simulink model "qpsk"  (R2015a)
settings: Solver=ode4  SolverMode=SingleTasking  StartTime=0.0  StopTime=Inf  RelTol=1e-3
libraries: dspsrcs4 x4, simulink x3, commrandsrc2 x1, commutil2 x1
settings Model: Creator=Artyom  LastModifiedBy=Artyom
settings OptimizationCC: BlockReduction=off  BooleanDataType=off
settings DebuggingCC: SaveWithParameterizedLinksMsg=none  UnderspecifiedInitializationDetection=Classic  MergeDetectMultiDrivingBlocksExec=none  SignalResolutionControl=TryResolveAllWithWarning
settings HardwareCC: TargetLongLongMode=on  TargetIntDivRoundTo=Zero  TargetEndianess=LittleEndian  TargetHWDeviceType=MATLAB Host  ProdEqTarget=off

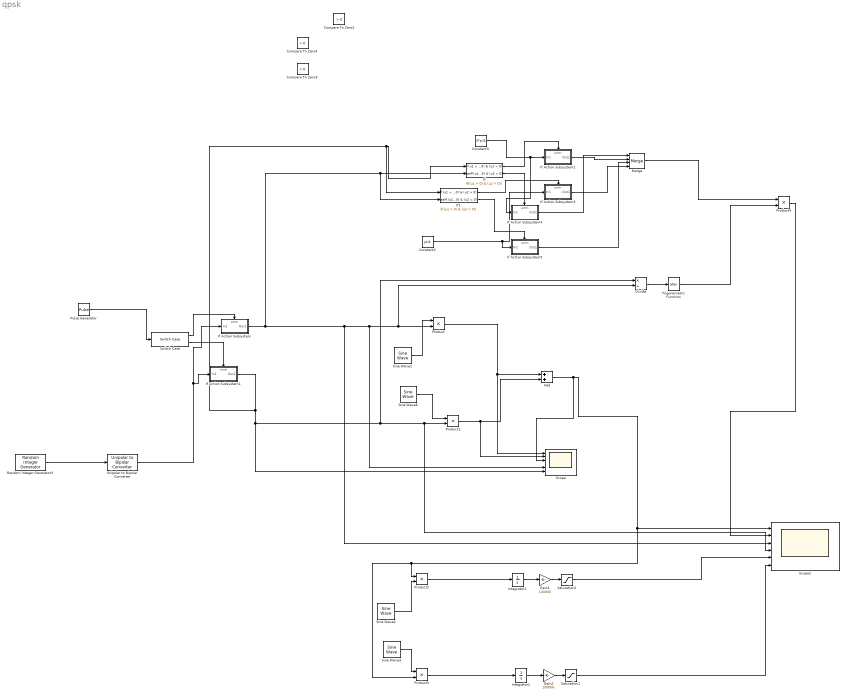
== system qpsk ==
  Add : Sum
  Compare To Zero2 : simulink/Logic and Bit Operations/Compare To Zero  relop=>  OutDataTypeStr=boolean
  Compare To Zero3 : simulink/Logic and Bit Operations/Compare To Zero  relop=<  OutDataTypeStr=boolean
  Compare To Zero4 : simulink/Logic and Bit Operations/Compare To Zero  relop=>  OutDataTypeStr=boolean
  Constant2 : Constant  Value=pi/4
  Constant3 : Constant  Value=3*pi/4
  Divide : Product  Inputs=*/
  Gain1 : Gain  Gain=100000
  Gain2 : Gain  Gain=100000
  If : If  NumInputs=2  IfExpression=(u1 < 0) & (u2 < 0)  ElseIfExpressions=(u1 < 0) & (u2 > 0)  ShowElse=off
  If Action Subsystem : Subsystem  TreatAsAtomicUnit=on
  If Action Subsystem1 : Subsystem  TreatAsAtomicUnit=on
  If Action Subsystem2 : Subsystem  TreatAsAtomicUnit=on
  If Action Subsystem3 : Subsystem  TreatAsAtomicUnit=on
  If Action Subsystem4 : Subsystem  TreatAsAtomicUnit=on
  If Action Subsystem5 : Subsystem  TreatAsAtomicUnit=on
  If1 : If  NumInputs=2  IfExpression=(u1 > 0) & (u2 > 0)  ElseIfExpressions=(u1 > 0) & (u2 < 0)  ShowElse=off
  Integrator1 : Integrator  LimitOutput=on  UpperSaturationLimit=0.00001  LowerSaturationLimit=-0.00001  ShowStatePort=on
  Integrator2 : Integrator  LimitOutput=on  UpperSaturationLimit=0.00001  LowerSaturationLimit=-0.00001  ShowStatePort=on
  Merge : Merge  Inputs=4
  Product : Product  OutDataTypeStr=Inherit: Same as first input
  Product{1..4} (4 alike) : Product
  Pulse Generator : DiscretePulseGenerator  PulseType=Time based  Period=1/5000  PulseWidth=50
  Random Integer Generator3 : commrandsrc2/Random Integer Generator  mul=2  seed=37  Ts=1/10000  frameBased=off  sampPerFrame=1  orient=on  outDataType=double
  Saturation1 : Saturate  UpperLimit=1  LowerLimit=-1
  Saturation2 : Saturate  UpperLimit=1  LowerLimit=-1
  Scope : Scope  NumInputPorts=6
      settings: YMin=-5~-5~-5~-5~-5~-5  YMax=5~5~5~5~5~5
  Scope2 : Scope  NumInputPorts=6
      settings: YMin=-0.00125~-5~-5~-5~-5~-5  YMax=0.00425~5~5~5~5~5  SaveName=ScopeData2
  Sine Wave1 : dspsrcs4/Sine Wave  Amplitude=1  Frequency=50000  Phase=pi/2  SampleMode=Discrete  OutComplex=Real  CompMethod=Trigonometric fcn  TableSize=Speed  SampleTime=1/1000000  SamplesPerFrame=1  ResetState=Restart at time zero  dataType=double  wordLen=16  udDataType=sfix(16)  fracBitsMode=Best precision  numFracBits=15  OutDataTypeStr=double  LastOutDataTypeStr=double
  Sine Wave2 : dspsrcs4/Sine Wave  Amplitude=1  Frequency=50000  Phase=pi/2  SampleMode=Discrete  OutComplex=Real  CompMethod=Trigonometric fcn  TableSize=Speed  SampleTime=1/1000000  SamplesPerFrame=1  ResetState=Restart at time zero  dataType=double  wordLen=16  udDataType=sfix(16)  fracBitsMode=Best precision  numFracBits=15  OutDataTypeStr=double  LastOutDataTypeStr=double
  Sine Wave3 : dspsrcs4/Sine Wave  Amplitude=1  Frequency=50000  Phase=0  SampleMode=Discrete  OutComplex=Real  CompMethod=Trigonometric fcn  TableSize=Speed  SampleTime=1/1000000  SamplesPerFrame=1  ResetState=Restart at time zero  dataType=double  wordLen=16  udDataType=sfix(16)  fracBitsMode=Best precision  numFracBits=15  OutDataTypeStr=double  LastOutDataTypeStr=double
  Sine Wave6 : dspsrcs4/Sine Wave  Amplitude=1  Frequency=50000  Phase=0  SampleMode=Discrete  OutComplex=Real  CompMethod=Trigonometric fcn  TableSize=Speed  SampleTime=1/1000000  SamplesPerFrame=1  ResetState=Restart at time zero  dataType=double  wordLen=16  udDataType=sfix(16)  fracBitsMode=Best precision  numFracBits=15  OutDataTypeStr=double  LastOutDataTypeStr=double
  Switch Case : SwitchCase  CaseConditions={1,0}  ShowDefaultCase=off
  Trigonometric Function : Trigonometry  Operator=atan  ApproximationMethod=CORDIC  OutputSignalType=real
  Unipolar to Bipolar Converter : commutil2/Unipolar to Bipolar Converter  M=2  polarity=Positive  dataType=Inherit via internal rule
  wires:
  Product/1 -> Scope/1, Add/1
  Sine Wave1/1 -> Product/1
  Sine Wave6/1 -> Product1/1
  Sine Wave2/1 -> Product2/2
  Sine Wave3/1 -> Product3/1
  Switch Case/1 -> If Action Subsystem/Action
  Pulse Generator/1 -> Switch Case/1
  Random Integer Generator3/1 -> Unipolar to Bipolar Converter/1
  Switch Case/2 -> If Action Subsystem1/Action
  Unipolar to Bipolar Converter/1 -> If Action Subsystem/1(In1), If Action Subsystem1/1(In1)
  Add/1 -> Scope/3, Scope2/1, Product3/2, Product2/1
  Product1/1 -> Scope/2, Add/2
  Divide/1 -> Trigonometric Function/1
  Trigonometric Function/1 -> Product4/2
  If Action Subsystem3/1(Out1) -> Merge/4
  If Action Subsystem/1(Out1) -> If/2, If1/2, Scope2/3, Scope/5, Divide/2, Product/2
  If/1 -> If Action Subsystem2/Action
  If1/1 -> If Action Subsystem3/Action
  If Action Subsystem5/1(Out1) -> Merge/3
  If/2 -> If Action Subsystem4/Action
  If1/2 -> If Action Subsystem5/Action
  Constant3/1 -> If Action Subsystem4/1(In1), If Action Subsystem2/1(In1)
  Constant2/1 -> If Action Subsystem5/1(In1), If Action Subsystem3/1(In1)
  If Action Subsystem2/1(Out1) -> Merge/2
  If Action Subsystem4/1(Out1) -> Merge/1
  Merge/1 -> Product4/1
  Product4/1 -> Scope2/2
  Integrator1/1 -> Gain1/1
  Gain1/1 -> Saturation2/1
  Product2/1 -> Integrator1/1
  Integrator2/1 -> Gain2/1
  Gain2/1 -> Saturation1/1
  Saturation1/1 -> Scope2/6
  Product3/1 -> Integrator2/1
  Saturation2/1 -> Scope2/5
  If Action Subsystem1/1(Out1) -> If1/1, If/1, Divide/1, Scope2/4, Product1/2, Scope/6

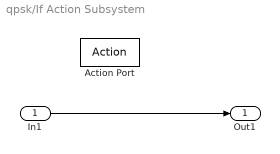
== system qpsk/If Action Subsystem ==
  In1 : Inport
  Action Port : ActionPort  ActionType=case
  Out1 : Outport
  wires:
  In1/1 -> Out1/1

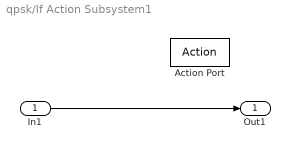
== system qpsk/If Action Subsystem1 ==
  In1 : Inport
  Action Port : ActionPort  ActionType=case
  Out1 : Outport
  wires:
  In1/1 -> Out1/1

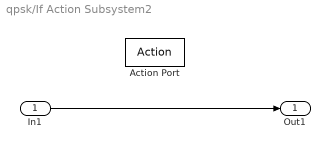
== system qpsk/If Action Subsystem2 ==
  In1 : Inport
  Action Port : ActionPort  ActionType=then
  Out1 : Outport
  wires:
  In1/1 -> Out1/1

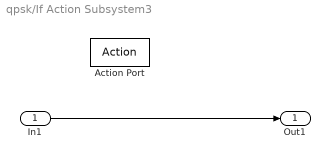
== system qpsk/If Action Subsystem3 ==
  In1 : Inport
  Action Port : ActionPort  ActionType=then
  Out1 : Outport
  wires:
  In1/1 -> Out1/1

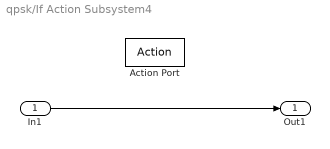
== system qpsk/If Action Subsystem4 ==
  In1 : Inport
  Action Port : ActionPort  ActionType=elseif
  Out1 : Outport
  wires:
  In1/1 -> Out1/1

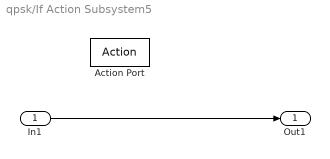
== system qpsk/If Action Subsystem5 ==
  In1 : Inport
  Action Port : ActionPort  ActionType=elseif
  Out1 : Outport
  wires:
  In1/1 -> Out1/1
